simulink model "asgnmnt5"  (R2018a)
settings: Solver=ode45  StartTime=0.0  StopTime=10.0  RelTol=1e-7
settings Model: Creator=ewk15101  LastModifiedBy=ewk15101

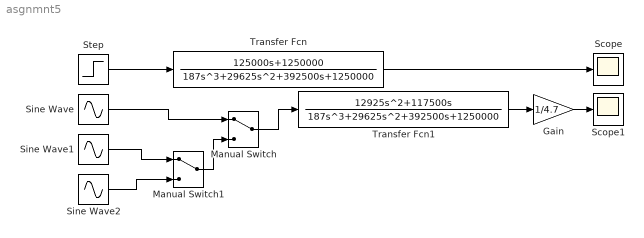
== system asgnmnt5 ==
  Gain : Gain  Gain=1/4.7
  Manual Switch : ManualSwitch
  Manual Switch1 : ManualSwitch
  Scope : Scope
  Scope1 : Scope
  Sine Wave : Sin  Frequency=2  SampleTime=0
  Sine Wave1 : Sin  Frequency=30  SampleTime=0
  Sine Wave2 : Sin  Frequency=200  SampleTime=0
  Step : Step  SampleTime=0
  Transfer Fcn : TransferFcn  Numerator=[125000 1250000]  Denominator=[187 29625 392500 1250000]
  Transfer Fcn1 : TransferFcn  Numerator=[12925 117500 0]  Denominator=[187 29625 392500 1250000]
  wires:
  Transfer Fcn/1 -> Scope/1
  Step/1 -> Transfer Fcn/1
  Sine Wave1/1 -> Manual Switch1/1
  Sine Wave2/1 -> Manual Switch1/2
  Sine Wave/1 -> Manual Switch/1
  Manual Switch1/1 -> Manual Switch/2
  Manual Switch/1 -> Transfer Fcn1/1
  Gain/1 -> Scope1/1
  Transfer Fcn1/1 -> Gain/1
